simulink model "aadc_1p5b"  (R2018b)
settings: Solver=FixedStepAuto  StartTime=0.0  StopTime=5000*2.2*2  FixedStep=1  RelTol=1e-3
libraries: simulink x2, dspswit3 x1, simulink_extras x1
settings Model: PauseTimes=66  Creator=anton  LastModifiedBy=anton
settings DataIOCC: SaveOutput=off  SignalLogging=off  DSMLogging=off  SaveTime=off
settings DebuggingCC: ReadBeforeWriteMsg=DisableAll  WriteAfterWriteMsg=DisableAll  WriteAfterReadMsg=DisableAll  MultiTaskDSMMsg=none
settings ModelReferenceCC: UpdateModelReferenceTargets=IfOutOfDate
settings SFSimCC: SFSimEcho=off

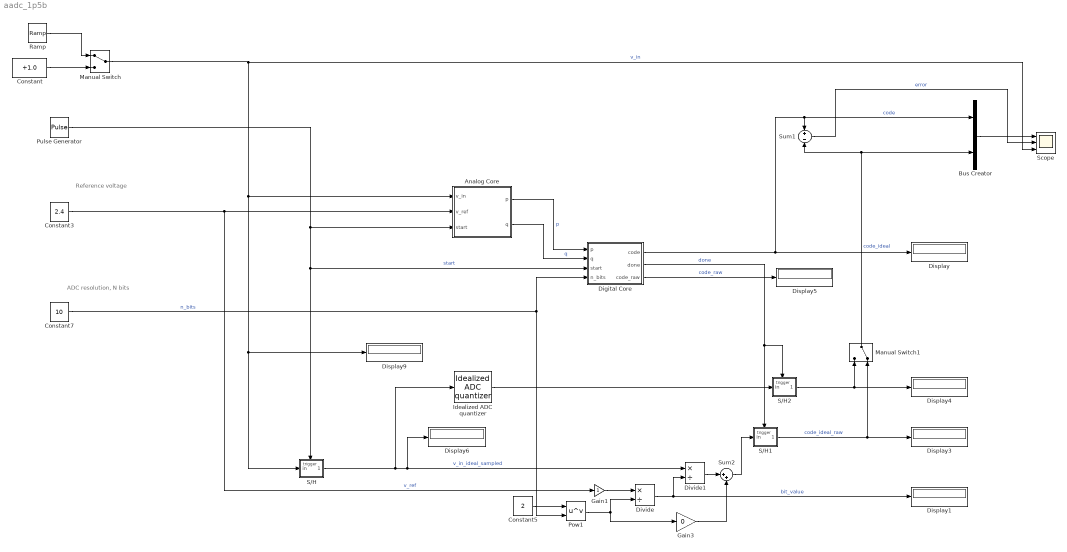
== system aadc_1p5b ==
  note: Reference voltage
  note: ADC resolution, N bits
  Analog Core : Subsystem
  Bus Creator : BusCreator  Inputs=2
  Constant : Constant  Value=+1.0
  Constant3 : Constant  Value=2.4
  Constant5 : Constant  Value=2
  Constant7 : Constant  Value=10
  Digital Core : Subsystem
  Display{,1,3..6,9} (7 alike) : Display
  Divide : Product  Inputs=*/
  Divide1 : Product  Inputs=*/
  Gain1 : Gain
  Gain3 : Gain  Gain=0
  Idealized ADC quantizer : simulink_extras/Additional Discrete/Idealized ADC quantizer  NumberOfConverterBits=11  Vmin=-2.4  Vmax=2.4  OutputDataType=double  OutputNegativeValues=on
      settings: SourceProductName=Simulink
  Manual Switch : ManualSwitch
  Manual Switch1 : ManualSwitch  CurrentSetting=0
  Pow1 : Math  Operator=pow  RndMeth=Zero  SaturateOnIntegerOverflow=on
  Pulse Generator : DiscretePulseGenerator  Period=11  PhaseDelay=1
  Ramp : simulink/Sources/Ramp  slope=(0.00234375/11)/1  start=1  InitialOutput=-2.4
  S/H : Subsystem
  S/H1 : Subsystem
  S/H2 : Subsystem
  Scope : Scope  NumInputPorts=3
  Sum1 : Sum  Inputs=+-
  Sum2 : Sum  Inputs=|++
  wires:
  Manual Switch/1 -> Scope/3, Display9/1, S/H/1(in), Analog Core/1(v_in)  "v_in"
  Constant3/1 -> Gain1/1, Analog Core/2(v_ref)  "v_ref"
  Pulse Generator/1 -> S/H/Trigger, Digital Core/3(start), Analog Core/3(start)  "start"
  Constant7/1 -> Digital Core/4(n_bits), Pow1/2  "n_bits"
  Gain1/1 -> Divide/1
  Pow1/1 -> Divide/2, Gain3/1
  Divide/1 -> Divide1/2, Display1/1  "bit_value"
  Gain3/1 -> Sum2/2
  Divide1/1 -> Sum2/1
  Constant5/1 -> Pow1/1
  Digital Core/1(code) -> Sum1/1, Bus Creator/1, Display/1  "code"
  Digital Core/2(done) -> S/H2/Trigger, S/H1/Trigger  "done"
  Analog Core/1(p) -> Digital Core/1(p)  "p"
  S/H2/1(out) -> Manual Switch1/1, Display4/1
  Digital Core/3(code_raw) -> Display5/1  "code_raw"
  Sum1/1 -> Scope/2  "error"
  S/H/1(out) -> Idealized ADC quantizer/1, Display6/1, Divide1/1  "v_in_ideal_sampled"
  S/H1/1(out) -> Manual Switch1/2, Display3/1  "code_ideal_raw"
  Sum2/1 -> S/H1/1(in)
  Bus Creator/1 -> Scope/1
  Constant/1 -> Manual Switch/2
  Ramp/1 -> Manual Switch/1
  Analog Core/2(q) -> Digital Core/2(q)  "q"
  Manual Switch1/1 -> Sum1/2, Bus Creator/2  "code_ideal"
  Idealized ADC quantizer/1 -> S/H2/1(in)

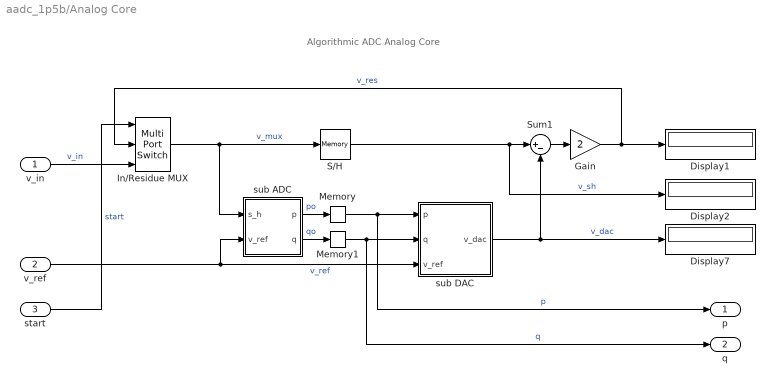
== system aadc_1p5b/Analog Core ==
  note: Algorithmic ADC Analog Core
  v_in : Inport
  v_ref : Inport  Port=2
  start : Inport  Port=3
  Display1 : Display
  Display2 : Display
  Display7 : Display
  Gain : Gain  Gain=2
  In/Residue MUX : MultiPortSwitch  DataPortOrder=Zero-based contiguous  Inputs=2  zeroidx=on
  Memory : Memory
  Memory1 : Memory
  S/H : Memory
  Sum1 : Sum  Inputs=|+-
  sub ADC : Subsystem
      mask Display: image('adc.png');
  sub DAC : Subsystem
      mask Display: image('dac.png');
  p : Outport
  q : Outport  Port=2
  wires:
  start/1 -> In/Residue MUX/1  "start"
  v_ref/1 -> sub DAC/3(v_ref), sub ADC/2(v_ref)  "v_ref"
  sub DAC/1(v_dac) -> Sum1/2, Display7/1  "v_dac"
  sub ADC/1(p) -> Memory/1  "po"
  Sum1/1 -> Gain/1
  v_in/1 -> In/Residue MUX/3  "v_in"
  Gain/1 -> In/Residue MUX/2, Display1/1  "v_res"
  In/Residue MUX/1 -> S/H/1, sub ADC/1(s_h)  "v_mux"
  sub ADC/2(q) -> Memory1/1  "qo"
  S/H/1 -> Display2/1, Sum1/1  "v_sh"
  Memory/1 -> p/1, sub DAC/1(p)  "p"
  Memory1/1 -> q/1, sub DAC/2(q)  "q"

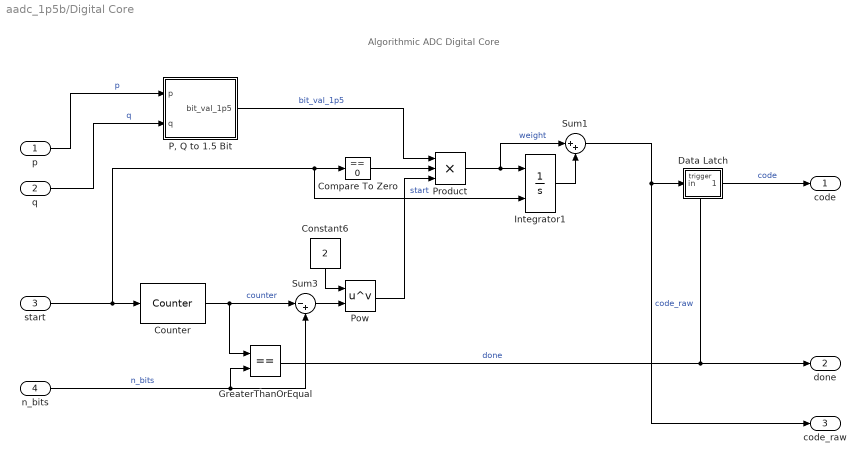
== system aadc_1p5b/Digital Core ==
  note: Algorithmic ADC Digital Core
  p : Inport
  q : Inport  Port=2
  start : Inport  Port=3
  n_bits : Inport  Port=4
  Compare To Zero : simulink/Logic and Bit Operations/Compare To Zero  relop===  OutDataTypeStr=boolean
  Constant6 : Constant  Value=2
  Counter : dspswit3/Counter  Direction=Up  CountEvent=Free running  CounterSize=32 bits  MaxCount=255  InitialCount=0  Output=Count  HitValue=32  ResetInput=on  SamplesPerFrame=1  Ts=-1  CntDtype=double  HitDtype=Logical
  Data Latch : Subsystem
  GreaterThanOrEqual : RelationalOperator  Operator===  OutDataTypeStr=boolean  RndMeth=Simplest
  Integrator1 : Integrator  ExternalReset=level
  "P, Q to 1.5 Bit" : MATLAB Function  TreatAsAtomicUnit=on
  Pow : Math  Operator=pow  RndMeth=Zero  SaturateOnIntegerOverflow=on
  Product : Product  Inputs=3
  Sum1 : Sum  Inputs=|++
  Sum3 : Sum  Inputs=|-+
  code : Outport
  done : Outport  Port=2
  code_raw : Outport  Port=3
  wires:
  n_bits/1 -> Sum3/2, GreaterThanOrEqual/2  "n_bits"
  start/1 -> Integrator1/2, Compare To Zero/1, Counter/1  "start"
  Sum3/1 -> Pow/2
  "P, Q to 1.5 Bit"/1(bit_val_1p5) -> Product/1  "bit_val_1p5"
  Product/1 -> Sum1/1, Integrator1/1  "weight"
  Pow/1 -> Product/3
  Counter/1 -> GreaterThanOrEqual/1, Sum3/1  "counter"
  Compare To Zero/1 -> Product/2
  Constant6/1 -> Pow/1
  GreaterThanOrEqual/1 -> Data Latch/Trigger, done/1  "done"
  Data Latch/1(out) -> code/1  "code"
  Sum1/1 -> Data Latch/1(in), code_raw/1  "code_raw"
  Integrator1/1 -> Sum1/2
  p/1 -> "P, Q to 1.5 Bit"/1(p)  "p"
  q/1 -> "P, Q to 1.5 Bit"/2(q)  "q"

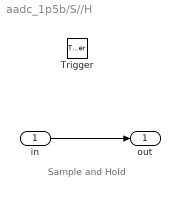
== system aadc_1p5b/S//H ==
  note: Sample and Hold
  in : Inport
  Trigger : TriggerPort  VariantControl=Variant  InitialTriggerSignalState=positive  PortDimensions=1
  out : Outport
  wires:
  in/1 -> out/1

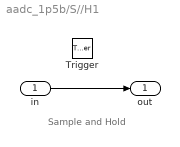
== system aadc_1p5b/S//H1 ==
  note: Sample and Hold
  in : Inport
  Trigger : TriggerPort  VariantControl=Variant  InitialTriggerSignalState=positive  PortDimensions=1
  out : Outport
  wires:
  in/1 -> out/1

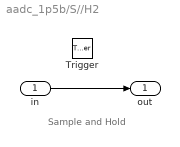
== system aadc_1p5b/S//H2 ==
  note: Sample and Hold
  in : Inport
  Trigger : TriggerPort  VariantControl=Variant  InitialTriggerSignalState=positive  PortDimensions=1
  out : Outport
  wires:
  in/1 -> out/1

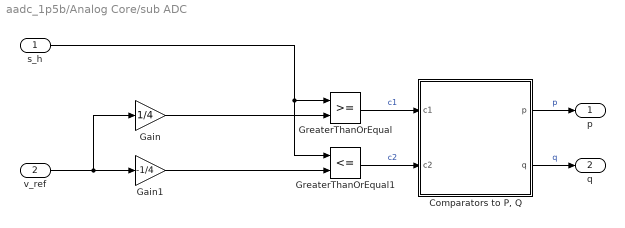
== system aadc_1p5b/Analog Core/sub ADC ==
  s_h : Inport
  v_ref : Inport  Port=2
  "Comparators to P, Q" : MATLAB Function  TreatAsAtomicUnit=on
  Gain : Gain  Gain=1/4
  Gain1 : Gain  Gain=-1/4
  GreaterThanOrEqual : RelationalOperator  OutDataTypeStr=boolean  RndMeth=Simplest
  GreaterThanOrEqual1 : RelationalOperator  Operator=<=  OutDataTypeStr=boolean  RndMeth=Simplest
  p : Outport
  q : Outport  Port=2
  wires:
  "Comparators to P, Q"/1(p) -> p/1  "p"
  s_h/1 -> GreaterThanOrEqual1/1, GreaterThanOrEqual/1
  "Comparators to P, Q"/2(q) -> q/1  "q"
  Gain1/1 -> GreaterThanOrEqual1/2
  Gain/1 -> GreaterThanOrEqual/2
  v_ref/1 -> Gain1/1, Gain/1
  GreaterThanOrEqual/1 -> "Comparators to P, Q"/1(c1)  "c1"
  GreaterThanOrEqual1/1 -> "Comparators to P, Q"/2(c2)  "c2"

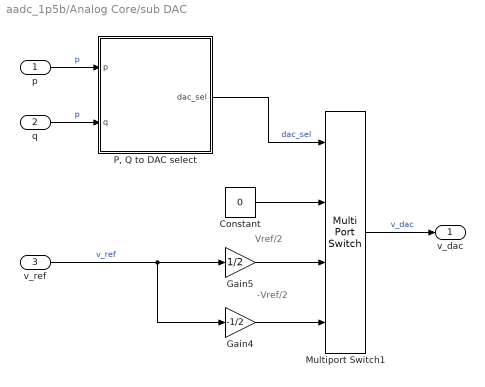
== system aadc_1p5b/Analog Core/sub DAC ==
  note: Vref/2
  note: -Vref/2
  p : Inport
  q : Inport  Port=2
  v_ref : Inport  Port=3
  Constant : Constant  Value=0
  Gain4 : Gain  Gain=-1/2
  Gain5 : Gain  Gain=1/2
  Multiport Switch1 : MultiPortSwitch  DataPortOrder=Zero-based contiguous  zeroidx=on
  "P, Q to DAC select" : MATLAB Function  TreatAsAtomicUnit=on
  v_dac : Outport
  wires:
  v_ref/1 -> Gain4/1, Gain5/1  "v_ref"
  Multiport Switch1/1 -> v_dac/1  "v_dac"
  Gain4/1 -> Multiport Switch1/4
  p/1 -> "P, Q to DAC select"/1(p)  "p"
  Gain5/1 -> Multiport Switch1/3
  q/1 -> "P, Q to DAC select"/2(q)  "p"
  "P, Q to DAC select"/1(dac_sel) -> Multiport Switch1/1  "dac_sel"
  Constant/1 -> Multiport Switch1/2

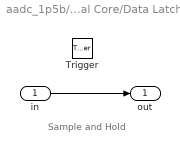
== system aadc_1p5b/Digital Core/Data Latch ==
  note: Sample and Hold
  in : Inport
  Trigger : TriggerPort  VariantControl=Variant  PortDimensions=1
  out : Outport
  wires:
  in/1 -> out/1

== matlab function aadc_1p5b/Analog Core/sub DAC/P, Q to DAC select ==
  data: p input; dac_sel output; q input
function dac_sel = fcn(p, q)
    dac_sel=0;
    if p==1 && q==0
        % Vin>=Vref/4
        dac_sel=1;% -Vref
    elseif p==0 && q==1
        % Vin<=-Vref/4
        dac_sel=2;% +Vref
    elseif p==0 && q==0
        % -Vref/4<Vin<Vref/4
        dac_sel=0;% 0*Vref
    end

== matlab function aadc_1p5b/Analog Core/sub ADC/Comparators to P, Q ==
  data: c1 input; p output; c2 input; q output
function [p, q] = fcn(c1, c2)
    p=0; q=0;
    if c1==1
        % Vin>=Vref/4
        p=1; q=0;
    elseif c2==1
        % Vin<=-Vref/4
        p=0; q=1;
    elseif c1==0 && c2==0
        % -Vref/4<Vin<Vref/4
        p=0; q=0;
    end

== matlab function aadc_1p5b/Digital Core/P, Q to 1.5 Bit ==
  data: p input; bit_val_1p5 output; q input
function bit_val_1p5 = fcn(p, q)
    bit_val_1p5=0;
    if p==1 && q==0
        % Vin>=Vref/4
        bit_val_1p5=+1;% -Vref
    elseif p==0 && q==1
        % Vin<=-Vref/4
        bit_val_1p5=-1;% +Vref
    elseif p==0 && q==0
        % -Vref/4<Vin<Vref/4
        bit_val_1p5=0;% 0*Vref
    end
